simulink model "Bicycle_Model"  (R2024a)
settings: Solver=FixedStepAuto  StartTime=0.0  StopTime=10.0  FixedStep=0.01  RelTol=1e-3
values from neighbouring files (symbols this model uses):
  a = 1.8    [BModel_Parameters.m]    (also in Longitudinal_Braking_Parameters.m)
  A = 1.25    [BModel_Parameters.m]    (also in Longitudinal_Braking_Parameters.m)
  a1f = -1e-5    (= -1e-05)    [BModel_Parameters.m]
  a1r = -1e-5    (= -1e-05)    [BModel_Parameters.m]
  a2f = 1.25    [BModel_Parameters.m]
  a2r = 1.25    [BModel_Parameters.m]
  b = L-a    (= 1.7)    [BModel_Parameters.m]    (also in Longitudinal_Braking_Parameters.m)
  Bf = 0.2719    [BModel_Parameters.m]
  Br = 0.3609    [BModel_Parameters.m]
  Cf = 1.8391    [BModel_Parameters.m]
  Cr = 1.7631    [BModel_Parameters.m]
  cz = 1    [BModel_Parameters.m]    (also in Longitudinal_Braking_Parameters.m)
  Ef = -2.5276    [BModel_Parameters.m]
  Er = -1.9890    (= -1.989)    [BModel_Parameters.m]
  g = 9.81    [BModel_Parameters.m]    (also in Longitudinal_Braking_Parameters.m)
  I = 1500    [BModel_Parameters.m]
  L = 3.5    [BModel_Parameters.m]    (also in Longitudinal_Braking_Parameters.m)
  m = 850    [BModel_Parameters.m]    (also in Longitudinal_Braking_Parameters.m)
  rho = 1.225    [BModel_Parameters.m]    (also in Longitudinal_Braking_Parameters.m)
  SR = 10    [BModel_Parameters.m]
libraries: simulink_extras x5
settings Model: Creator=gaurimorjaria  LastModifiedBy=gaurimorjaria

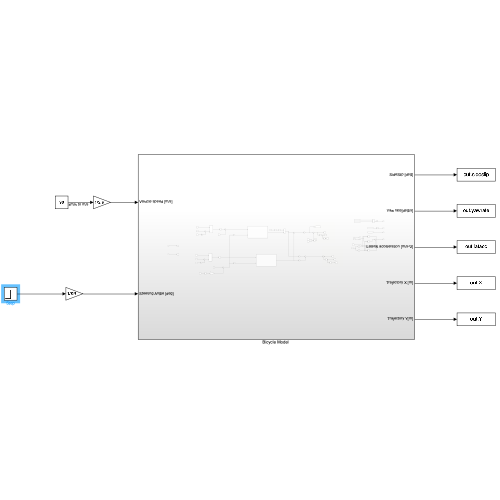
[thumbnail: Simulink's stored preview of the top-level diagram]
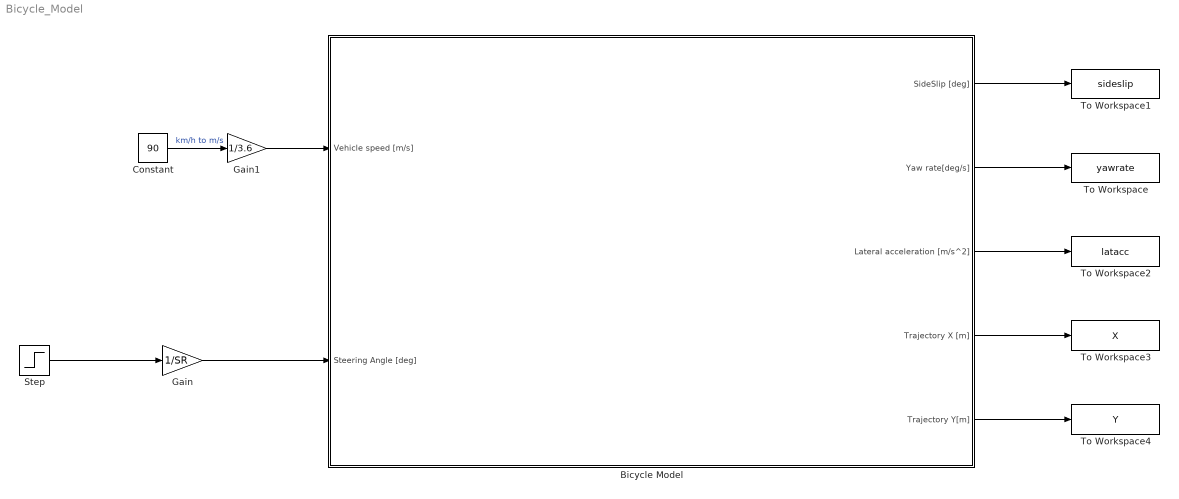
== system Bicycle_Model ==
  "Bicycle Model " : Subsystem
  Constant : Constant  Value=90
  Gain : Gain  Gain=1/SR
  Gain1 : Gain  Gain=1/3.6
  Step : Step  Time=3  After=10  SampleTime=0
  To Workspace : ToWorkspace  VariableName=yawrate  SaveFormat=Timeseries  SampleTime=-1
  To Workspace1 : ToWorkspace  VariableName=sideslip  SampleTime=-1
  To Workspace2 : ToWorkspace  VariableName=latacc  SaveFormat=Timeseries  SampleTime=-1
  To Workspace3 : ToWorkspace  VariableName=X  SaveFormat=Timeseries  SampleTime=-1
  To Workspace4 : ToWorkspace  VariableName=Y  SaveFormat=Timeseries  SampleTime=-1
  wires:
  "Bicycle Model "/1(SideSlip [deg]) -> To Workspace1/1
  "Bicycle Model "/5(Trajectory Y[m]) -> To Workspace4/1
  "Bicycle Model "/4(Trajectory X [m]) -> To Workspace3/1
  "Bicycle Model "/3(Lateral acceleration [m/s^2]) -> To Workspace2/1
  "Bicycle Model "/2(Yaw rate[deg/s]) -> To Workspace/1
  Gain/1 -> "Bicycle Model "/2(Steering Angle [deg])
  Gain1/1 -> "Bicycle Model "/1(Vehicle speed [m/s])
  Constant/1 -> Gain1/1  "km/h to m/s"
  Step/1 -> Gain/1

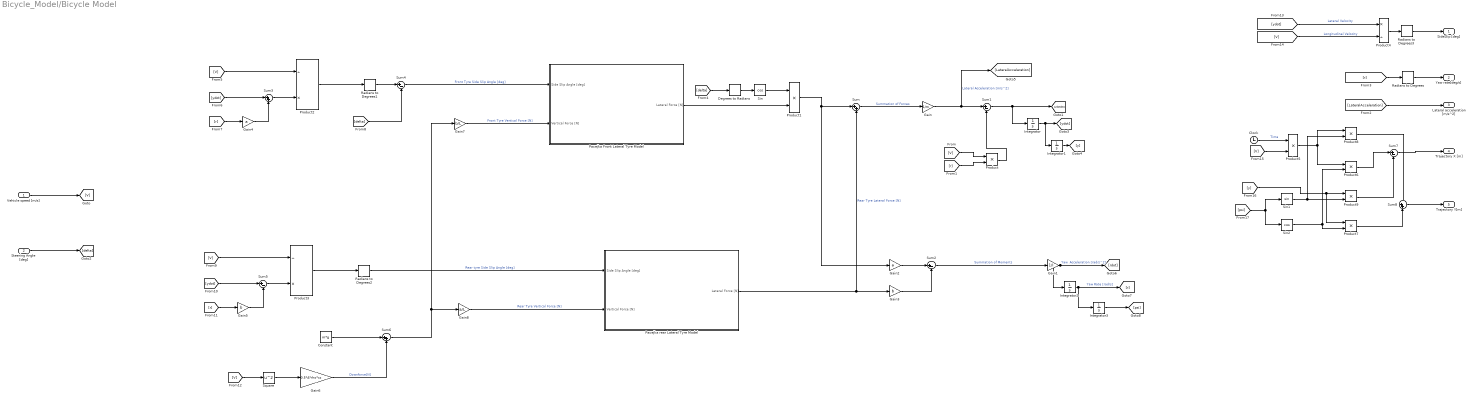
== system Bicycle_Model/Bicycle Model  ==
  Vehicle speed [m/s] : Inport
  Steering Angle [deg] : Inport  Port=2
  Clock : Clock
  Constant : Constant  Value=m*g
  Degrees to Radians : simulink_extras/Transformations/Degrees to Radians
  Gain : Gain  Gain=1/m
  Gain1 : Gain  Gain=1/I
  Gain2 : Gain  Gain=a
  Gain3 : Gain  Gain=b
  Gain4 : Gain  Gain=a
  Gain5 : Gain  Gain=b
  Gain6 : Gain  Gain=0.5*A*rho*cz
  Gain7 : Gain  Gain=b/L
  Gain8 : Gain  Gain=a/L
  Integrator{,1..3} (4 alike) : Integrator
  Pacejka Front Lateral Tyre Model : Subsystem
  Pacejka rear Lateral Tyre Model : Subsystem
  Product{,1,5..9} (7 alike) : Product
  Product2 : Product  Inputs=/*
  Product3 : Product  Inputs=/*
  Product4 : Product  Inputs=*/
  Radians to Degrees{,1..3} (4 alike) : simulink_extras/Transformations/Radians to Degrees
  Sin : Trigonometry  Operator=cos
  Sin1 : Trigonometry
  Sin2 : Trigonometry  Operator=cos
  Square : Math  Operator=square
  Sum{,3,6,8} (4 alike) : Sum  Inputs=|++
  Sum{1..2,4..5,7} (5 alike) : Sum  Inputs=|+-
  SideSlip [deg] : Outport
  Yaw rate[deg/s] : Outport  Port=2
  Lateral acceleration [m/s^2] : Outport  Port=3
  Trajectory X [m] : Outport  Port=4
  Trajectory Y[m] : Outport  Port=5
  wires:
  Vehicle speed [m/s]/1 -> [V]
  Sum/1 -> Gain/1  "Summation of Forces"
  Gain/1 -> [LateralAcceleration], Sum1/1  "Lateral Acceleration [m/s^2]"
  Product/1 -> Sum1/2
  [r] -> Product/2
  [V] -> Product/1
  Sum1/1 -> Integrator/1, [ydotdot]
  Integrator/1 -> Integrator1/1, [ydot]
  Integrator1/1 -> [y]
  [LateralAcceleration] -> Lateral acceleration [m/s^2]/1
  Sum2/1 -> Gain1/1  "Summation of Moments"
  Gain1/1 -> Integrator2/1, [rdot]  "Yaw  Acceleration [rad/s^2]"
  Integrator2/1 -> [r], Integrator3/1  "Yaw Rate [rad/s]"
  Integrator3/1 -> [psi]
  [r] -> Radians to Degrees/1
  Radians to Degrees/1 -> Yaw rate[deg/s]/1
  Gain2/1 -> Sum2/1
  Gain3/1 -> Sum2/2
  Pacejka rear Lateral Tyre Model/1(Lateral Force [N]) -> Sum/2, Gain3/1  "Rear Tyre Lateral Force [N]"
  Pacejka Front Lateral Tyre Model/1(Lateral Force [N]) -> Product1/2
  Product1/1 -> Gain2/1, Sum/1
  [delta] -> Degrees to Radians/1
  Degrees to Radians/1 -> Sin/1
  Sin/1 -> Product1/1
  Sum3/1 -> Product2/2
  [V] -> Product2/1
  [ydot] -> Sum3/1
  Gain4/1 -> Sum3/2
  [r] -> Gain4/1
  Product2/1 -> Radians to Degrees1/1
  Steering Angle [deg]/1 -> [delta]
  [delta] -> Sum4/2
  Radians to Degrees1/1 -> Sum4/1
  Sum4/1 -> Pacejka Front Lateral Tyre Model/1(Side Slip Angle [deg])  "Front Tyre Side Slip Angle [deg]"
  [V] -> Product3/1
  [ydot] -> Sum5/1
  Gain5/1 -> Sum5/2
  [r] -> Gain5/1
  Product3/1 -> Radians to Degrees2/1
  Sum5/1 -> Product3/2
  Radians to Degrees2/1 -> Pacejka rear Lateral Tyre Model/1(Side Slip Angle [deg])  "Rear tyre Side Slip Angle [deg]"
  Constant/1 -> Sum6/1
  [V] -> Square/1
  Square/1 -> Gain6/1
  Gain6/1 -> Sum6/2  "Downforce[N]"
  Gain7/1 -> Pacejka Front Lateral Tyre Model/2(Vertical Force [N])  "Front Tyre Vertical Force [N]"
  Sum6/1 -> Gain7/1, Gain8/1
  Gain8/1 -> Pacejka rear Lateral Tyre Model/2(Vertical Force [N])  "Rear Tyre Vertical Force [N]"
  [ydot] -> Product4/1  "Lateral Velocity"
  [V] -> Product4/2  "Longitudinal Velocity"
  Product4/1 -> Radians to Degrees3/1
  Radians to Degrees3/1 -> SideSlip [deg]/1
  [V] -> Product5/2
  Clock/1 -> Product5/1  "Time"
  [psi] -> Sin2/1, Sin1/1
  Product5/1 -> Product6/1, Product8/1
  Sin1/1 -> Product8/2, Product9/2
  Sin2/1 -> Product7/2, Product6/2
  [y] -> Product7/1, Product9/1
  Sum7/1 -> Trajectory X [m]/1
  Sum8/1 -> Trajectory Y[m]/1
  Product9/1 -> Sum7/2
  Product6/1 -> Sum7/1
  Product8/1 -> Sum8/1
  Product7/1 -> Sum8/2

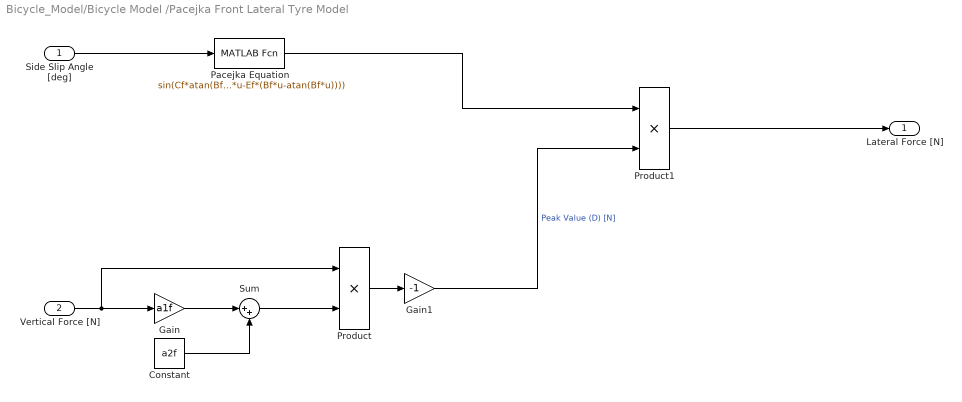
== system Bicycle_Model/Bicycle Model /Pacejka Front Lateral Tyre Model ==
  Side Slip Angle [deg] : Inport
  Vertical Force [N] : Inport  Port=2
  Constant : Constant  Value=a2f
  Gain : Gain  Gain=a1f
  Gain1 : Gain  Gain=-1
  Pacejka Equation : MATLABFcn  MATLABFcn=sin(Cf*atan(Bf*u-Ef*(Bf*u-atan(Bf*u))))
  Product : Product
  Product1 : Product
  Sum : Sum  Inputs=|++
  Lateral Force [N] : Outport
  wires:
  Vertical Force [N]/1 -> Product/1, Gain/1
  Gain/1 -> Sum/1
  Constant/1 -> Sum/2
  Sum/1 -> Product/2
  Product/1 -> Gain1/1
  Gain1/1 -> Product1/2  "Peak Value (D) [N]"
  Product1/1 -> Lateral Force [N]/1
  Side Slip Angle [deg]/1 -> Pacejka Equation/1
  Pacejka Equation/1 -> Product1/1

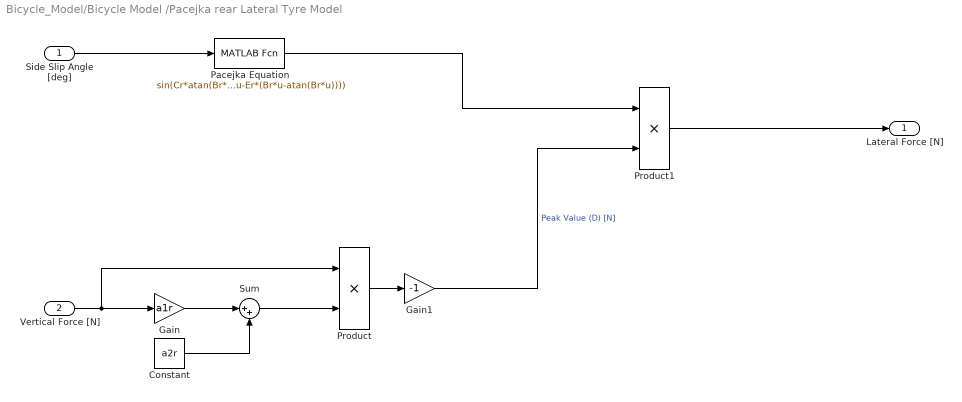
== system Bicycle_Model/Bicycle Model /Pacejka rear Lateral Tyre Model ==
  Side Slip Angle [deg] : Inport
  Vertical Force [N] : Inport  Port=2
  Constant : Constant  Value=a2r
  Gain : Gain  Gain=a1r
  Gain1 : Gain  Gain=-1
  Pacejka Equation : MATLABFcn  MATLABFcn=sin(Cr*atan(Br*u-Er*(Br*u-atan(Br*u))))
  Product : Product
  Product1 : Product
  Sum : Sum  Inputs=|++
  Lateral Force [N] : Outport
  wires:
  Pacejka Equation/1 -> Product1/1
  Side Slip Angle [deg]/1 -> Pacejka Equation/1
  Product1/1 -> Lateral Force [N]/1
  Gain1/1 -> Product1/2  "Peak Value (D) [N]"
  Product/1 -> Gain1/1
  Sum/1 -> Product/2
  Constant/1 -> Sum/2
  Gain/1 -> Sum/1
  Vertical Force [N]/1 -> Gain/1, Product/1
